simulink model "ddc_bpm_476_066"  (Simulink 7.8)
settings: Solver=ode45  StartTime=0.0  StopTime=2e-3  RelTol=1e-3
undefined symbols (not defined in the file): decim_factor_poly_35, dt_sim, frev_476, Fs_adc, n_ch, n_ovs, R_fofb, R_sec, R_sec_cfir, R_sec_pfir, xlipgetpartsetting
libraries: xbsIndex_r4 x1483, simulink x7
(part 11 of 12)

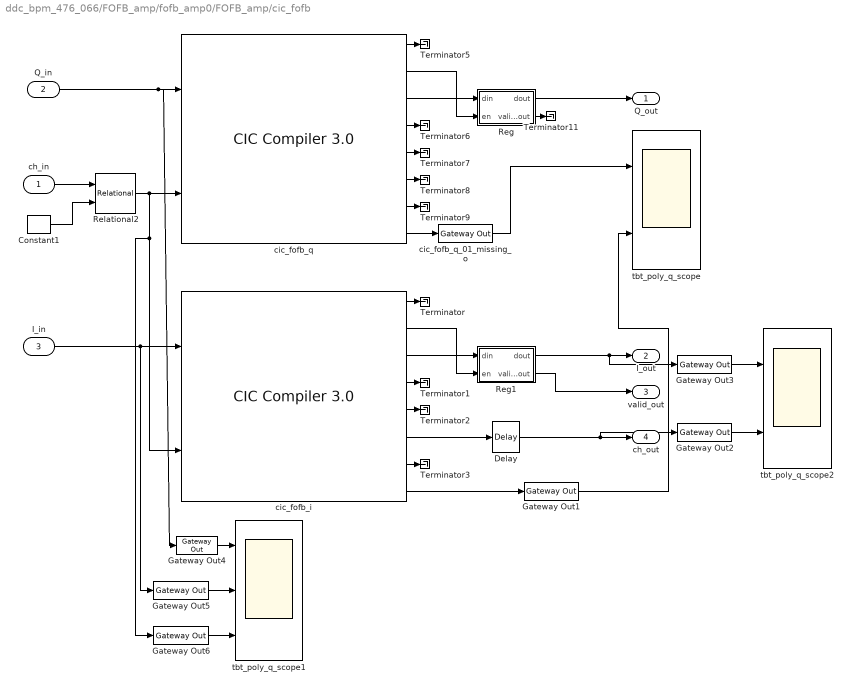
== system ddc_bpm_476_066/FOFB_amp/fofb_amp0/FOFB_amp/cic_fofb ==
  ch_in : Inport
  Q_in : Inport  Port=2
  I_in : Inport  Port=3
  Constant1 : xbsIndex_r4/Constant  const=0  gui_display_data_type=Fixed-point  arith_type=Unsigned  n_bits=2  bin_pt=0  preci_type=Single  exp_width=8  frac_width=24  explicit_period=off  period=1  equ=P=C  opselect=C  inp2=PCIN>>17  opr=+  inp1=P  carry=CIN  dbl_ovrd=off  block_type=constant
  Delay : xbsIndex_r4/Delay  rst=off  infoeditControl=Selection of Reset will increase slice count due to use of real FFs and instead of SRLs  en=off  latency=1  dbl_ovrd=off  reg_retiming=off  block_type=delay
  Gateway Out{1..6} (6 alike) : xbsIndex_r4/Gateway Out  inherit_from_input=on  hdl_port=off  timing_constraint=Data Rate  locs_specified=off  LOCs={}  UseAsDAC=off  DACChannel='1'  block_type=gatewayout
      settings: infoedit="Gateway out block.  Converts Xilinx fixed-point or floating-point type inputs into ouputs of type Simulink integer, single, double, or fixed point.<br><br>Hardware notes:  In hardware these blocks become top level output ports or are discarded, depending on how they are configured."
  Reg : Subsystem
  Reg1 : Subsystem
  Relational2 : xbsIndex_r4/Relational  mode=a=b  en=off  latency=1  dbl_ovrd=off  block_type=relational
  Terminator{,1..3,5..9,11} (10 alike) : Terminator
  cic_fofb_i : xbsIndex_r4/CIC Compiler 3.0   filter_type=Decimation  number_of_stages=5  differential_delay=2  number_of_channels=2  sample_rate_changes=Fixed  fixed_or_initial_rate=R_fofb  minimum_rate=1112  maximum_rate=1112  ratespecification=Maximum_Possible  sampleperiod=1  hardwareoversamplingrate=556  quantization=Full_Precision  output_data_width=74  use_xtreme_dsp_slice=on  use_streaming_interface=on  has_aclken=off  has_aresetn=off  has_dout_tready=off  trim_axipin_name=on  gui_behaviour=Sysgen_GUI  input_data_width=18  ip_name=CIC Compiler  ip_version=3.0  dsptool_ready=true  wrapper_available=true  port_translation_map={ 'aclken' => 'en', 'aresetn' => 'rst' }  ipcore_xco_need_fpga_part=true  ipcore_fpga_part=xlipgetpartsetting(gcb, {'virtex7', 'xc7v1500t', '-2', 'fhg1157'})  ipcore_verbose=false  block_type=cic_compiler_v3_0
  cic_fofb_q : xbsIndex_r4/CIC Compiler 3.0   filter_type=Decimation  number_of_stages=5  differential_delay=2  number_of_channels=2  sample_rate_changes=Fixed  fixed_or_initial_rate=R_fofb  minimum_rate=1112  maximum_rate=1112  ratespecification=Maximum_Possible  sampleperiod=1  hardwareoversamplingrate=556  quantization=Full_Precision  output_data_width=74  use_xtreme_dsp_slice=on  use_streaming_interface=on  has_aclken=off  has_aresetn=off  has_dout_tready=off  trim_axipin_name=on  gui_behaviour=Sysgen_GUI  input_data_width=18  ip_name=CIC Compiler  ip_version=3.0  dsptool_ready=true  wrapper_available=true  port_translation_map={ 'aclken' => 'en', 'aresetn' => 'rst' }  ipcore_xco_need_fpga_part=true  ipcore_fpga_part=xlipgetpartsetting(gcb, {'virtex7', 'xc7v1500t', '-2', 'fhg1157'})  ipcore_verbose=false  block_type=cic_compiler_v3_0
  cic_fofb_q_01_missing_o : xbsIndex_r4/Gateway Out  inherit_from_input=on  hdl_port=on  timing_constraint=Data Rate  locs_specified=off  LOCs={}  UseAsDAC=off  DACChannel='1'  block_type=gatewayout
      settings: infoedit="Gateway out block.  Converts Xilinx fixed-point or floating-point type inputs into ouputs of type Simulink integer, single, double, or fixed point.<br><br>Hardware notes:  In hardware these blocks become top level output ports or are discarded, depending on how they are configured."
  tbt_poly_q_scope : Scope  NumInputPorts=2
      settings: TimeRange=0.00011214  YMin=-0.1~-1.5  YMax=1~1.5  SaveName=ScopeData11  MaxDataPoints=1000000  SampleInput=on
  tbt_poly_q_scope1 : Scope  NumInputPorts=3
      settings: TimeRange=0.00011214  YMin=-0.1~-1.5~-5  YMax=1~1.5~5  SaveName=ScopeData12  MaxDataPoints=1000000  SampleInput=on
  tbt_poly_q_scope2 : Scope  NumInputPorts=2
      settings: TimeRange=0.00018  YMin=-5.05447e-005~0.9999999998750002  YMax=-5.05447e-005~1.000000000125  SaveName=ScopeData17  MaxDataPoints=1000000  SampleInput=on
  Q_out : Outport
  I_out : Outport  Port=2
  valid_out : Outport  Port=3
  ch_out : Outport  Port=4
  wires:
  I_in/1 -> cic_fofb_i/1, Gateway Out5/1
  Q_in/1 -> cic_fofb_q/1, Gateway Out4/1
  Relational2/1 -> cic_fofb_q/2, cic_fofb_i/2, Gateway Out6/1
  ch_in/1 -> Relational2/1
  cic_fofb_i/6 -> Delay/1
  cic_fofb_i/1 -> Terminator/1
  cic_fofb_i/4 -> Terminator1/1
  cic_fofb_i/5 -> Terminator2/1
  cic_fofb_i/7 -> Terminator3/1
  cic_fofb_q/1 -> Terminator5/1
  cic_fofb_q/4 -> Terminator6/1
  cic_fofb_q/5 -> Terminator7/1
  cic_fofb_q/6 -> Terminator8/1
  cic_fofb_q/7 -> Terminator9/1
  Constant1/1 -> Relational2/2
  Reg/1(dout) -> Q_out/1
  cic_fofb_q/3 -> Reg/1(din)
  cic_fofb_q/2 -> Reg/2(en)
  Reg1/1(dout) -> I_out/1, Gateway Out3/1
  cic_fofb_i/3 -> Reg1/1(din)
  cic_fofb_i/2 -> Reg1/2(en)
  Reg1/2(valid_out) -> valid_out/1
  Delay/1 -> ch_out/1, Gateway Out2/1
  Reg/2(valid_out) -> Terminator11/1
  cic_fofb_q/8 -> cic_fofb_q_01_missing_o/1
  cic_fofb_i/8 -> Gateway Out1/1
  cic_fofb_q_01_missing_o/1 -> tbt_poly_q_scope/1
  Gateway Out1/1 -> tbt_poly_q_scope/2
  Gateway Out2/1 -> tbt_poly_q_scope2/2
  Gateway Out3/1 -> tbt_poly_q_scope2/1
  Gateway Out4/1 -> tbt_poly_q_scope1/1
  Gateway Out5/1 -> tbt_poly_q_scope1/2
  Gateway Out6/1 -> tbt_poly_q_scope1/3

== system ddc_bpm_476_066/FOFB_amp/fofb_amp1/FOFB_CORDIC/TDDM_fofb_cordic1 ==
  fofb_cordic_din : Inport
  fofb_cordic_pin : Inport  Port=2
  fofb_cordic_ch_in : Inport  Port=3
  TDDM_fofb_cordic1_int : Subsystem
  TDDM_tbt_cordic1 : Subsystem
  Terminator : Terminator
  Terminator1 : Terminator
  fofb_cordic_data0_out : Outport
  fofb_cordic_data1_out : Outport  Port=2
  fofb_cordic_phase0_out : Outport  Port=3
  fofb_cordic_phase1_out : Outport  Port=4
  wires:
  TDDM_fofb_cordic1_int/2(dout_ch1) -> fofb_cordic_data1_out/1
  fofb_cordic_din/1 -> TDDM_fofb_cordic1_int/1(din)
  fofb_cordic_ch_in/1 -> TDDM_fofb_cordic1_int/2(ch_in), TDDM_tbt_cordic1/2(ch_in)
  TDDM_fofb_cordic1_int/1(dout_ch0) -> fofb_cordic_data0_out/1
  TDDM_fofb_cordic1_int/3(ch_out) -> Terminator/1
  TDDM_tbt_cordic1/2(dout_ch1) -> fofb_cordic_phase1_out/1
  fofb_cordic_pin/1 -> TDDM_tbt_cordic1/1(din)
  TDDM_tbt_cordic1/1(dout_ch0) -> fofb_cordic_phase0_out/1
  TDDM_tbt_cordic1/3(ch_out) -> Terminator1/1

== system ddc_bpm_476_066/FOFB_amp/fofb_amp1/FOFB_amp/Reg ==
  din : Inport
  Convert : xbsIndex_r4/Convert  gui_display_data_type=Fixed-point  arith_type="Signed  (2's comp)"  n_bits=24  bin_pt=22  float_type=Single  exp_bits=8  fraction_bits=24  quantization="Round  (unbiased: +/- Inf)"  overflow=Flag as error  en=off  latency=0  dbl_ovrd=off  pipeline=off  block_type=convert
  Register : xbsIndex_r4/Register  init=0  rst=off  en=off  dbl_ovrd=off  block_type=register
      settings: xl_area=[0, 0, 0, 0, 0, 0, 0]  block_version=VER_STRING_GOES_HERE
  Reinterpret2 : xbsIndex_r4/Reinterpret  force_arith_type=on  arith_type="Signed  (2's comp)"  force_bin_pt=on  bin_pt=23  block_type=cast
      settings: block_version=VER_STRING_GOES_HERE
  dout : Outport
  wires:
  Register/1 -> dout/1
  din/1 -> Reinterpret2/1
  Reinterpret2/1 -> Convert/1
  Convert/1 -> Register/1

== system ddc_bpm_476_066/FOFB_amp/fofb_amp1/FOFB_amp/Reg1 ==
  din : Inport
  Convert : xbsIndex_r4/Convert  gui_display_data_type=Fixed-point  arith_type="Signed  (2's comp)"  n_bits=24  bin_pt=22  float_type=Single  exp_bits=8  fraction_bits=24  quantization="Round  (unbiased: +/- Inf)"  overflow=Flag as error  en=off  latency=0  dbl_ovrd=off  pipeline=off  block_type=convert
  Register : xbsIndex_r4/Register  init=0  rst=off  en=off  dbl_ovrd=off  block_type=register
      settings: xl_area=[0, 0, 0, 0, 0, 0, 0]  block_version=VER_STRING_GOES_HERE
  Reinterpret2 : xbsIndex_r4/Reinterpret  force_arith_type=on  arith_type="Signed  (2's comp)"  force_bin_pt=on  bin_pt=23  block_type=cast
      settings: block_version=VER_STRING_GOES_HERE
  dout : Outport
  wires:
  Register/1 -> dout/1
  din/1 -> Reinterpret2/1
  Reinterpret2/1 -> Convert/1
  Convert/1 -> Register/1

== system ddc_bpm_476_066/FOFB_amp/fofb_amp1/FOFB_amp/TDDM_fofb_cic1 ==
  fofb_q_in : Inport
  fofb_i_in : Inport  Port=2
  fofb_ch_in : Inport  Port=3
  TDDM_fofb_cic1_i : Subsystem
  TDDM_fofb_cic1_q : Subsystem
  Terminator : Terminator
  Terminator1 : Terminator
  cic_fofb_ch0_q_out : Outport
  cic_fofb_ch1_q_out : Outport  Port=2
  cic_fofb_ch0_i_out : Outport  Port=3
  cic_fofb_ch1_i_out : Outport  Port=4
  wires:
  fofb_q_in/1 -> TDDM_fofb_cic1_q/1(din)
  fofb_ch_in/1 -> TDDM_fofb_cic1_q/2(ch_in), TDDM_fofb_cic1_i/2(ch_in)
  fofb_i_in/1 -> TDDM_fofb_cic1_i/1(din)
  TDDM_fofb_cic1_q/1(dout_ch0) -> cic_fofb_ch0_q_out/1
  TDDM_fofb_cic1_q/2(dout_ch1) -> cic_fofb_ch1_q_out/1
  TDDM_fofb_cic1_i/2(dout_ch1) -> cic_fofb_ch1_i_out/1
  TDDM_fofb_cic1_i/1(dout_ch0) -> cic_fofb_ch0_i_out/1
  TDDM_fofb_cic1_i/3(ch_out) -> Terminator/1
  TDDM_fofb_cic1_q/3(ch_out) -> Terminator1/1

== system ddc_bpm_476_066/FOFB_amp/fofb_amp1/FOFB_amp/cic_fofb ==
  ch_in : Inport
  Q_in : Inport  Port=2
  I_in : Inport  Port=3
  Constant1 : xbsIndex_r4/Constant  const=0  gui_display_data_type=Fixed-point  arith_type=Unsigned  n_bits=2  bin_pt=0  preci_type=Single  exp_width=8  frac_width=24  explicit_period=off  period=1  equ=P=C  opselect=C  inp2=PCIN>>17  opr=+  inp1=P  carry=CIN  dbl_ovrd=off  block_type=constant
  Delay : xbsIndex_r4/Delay  rst=off  infoeditControl=Selection of Reset will increase slice count due to use of real FFs and instead of SRLs  en=off  latency=1  dbl_ovrd=off  reg_retiming=off  block_type=delay
  Reg : Subsystem
  Reg1 : Subsystem
  Relational2 : xbsIndex_r4/Relational  mode=a=b  en=off  latency=1  dbl_ovrd=off  block_type=relational
  Terminator{,1..11} (12 alike) : Terminator
  cic_fofb_i : xbsIndex_r4/CIC Compiler 3.0   filter_type=Decimation  number_of_stages=5  differential_delay=2  number_of_channels=2  sample_rate_changes=Fixed  fixed_or_initial_rate=R_fofb  minimum_rate=1112  maximum_rate=1112  ratespecification=Maximum_Possible  sampleperiod=1  hardwareoversamplingrate=556  quantization=Full_Precision  output_data_width=74  use_xtreme_dsp_slice=on  use_streaming_interface=on  has_aclken=off  has_aresetn=off  has_dout_tready=off  trim_axipin_name=on  gui_behaviour=Sysgen_GUI  input_data_width=18  ip_name=CIC Compiler  ip_version=3.0  dsptool_ready=true  wrapper_available=true  port_translation_map={ 'aclken' => 'en', 'aresetn' => 'rst' }  ipcore_xco_need_fpga_part=true  ipcore_fpga_part=xlipgetpartsetting(gcb, {'virtex7', 'xc7v1500t', '-2', 'fhg1157'})  ipcore_verbose=false  block_type=cic_compiler_v3_0
  cic_fofb_q : xbsIndex_r4/CIC Compiler 3.0   filter_type=Decimation  number_of_stages=5  differential_delay=2  number_of_channels=2  sample_rate_changes=Fixed  fixed_or_initial_rate=R_fofb  minimum_rate=1112  maximum_rate=1112  ratespecification=Maximum_Possible  sampleperiod=1  hardwareoversamplingrate=556  quantization=Full_Precision  output_data_width=74  use_xtreme_dsp_slice=on  use_streaming_interface=on  has_aclken=off  has_aresetn=off  has_dout_tready=off  trim_axipin_name=on  gui_behaviour=Sysgen_GUI  input_data_width=18  ip_name=CIC Compiler  ip_version=3.0  dsptool_ready=true  wrapper_available=true  port_translation_map={ 'aclken' => 'en', 'aresetn' => 'rst' }  ipcore_xco_need_fpga_part=true  ipcore_fpga_part=xlipgetpartsetting(gcb, {'virtex7', 'xc7v1500t', '-2', 'fhg1157'})  ipcore_verbose=false  block_type=cic_compiler_v3_0
  cic_fofb_q_23_missing_o : xbsIndex_r4/Gateway Out  inherit_from_input=on  hdl_port=on  timing_constraint=Data Rate  locs_specified=off  LOCs={}  UseAsDAC=off  DACChannel='1'  block_type=gatewayout
      settings: infoedit="Gateway out block.  Converts Xilinx fixed-point or floating-point type inputs into ouputs of type Simulink integer, single, double, or fixed point.<br><br>Hardware notes:  In hardware these blocks become top level output ports or are discarded, depending on how they are configured."
  Q_out : Outport
  I_out : Outport  Port=2
  valid_out : Outport  Port=3
  ch_out : Outport  Port=4
  wires:
  I_in/1 -> cic_fofb_i/1
  Q_in/1 -> cic_fofb_q/1
  Relational2/1 -> cic_fofb_q/2, cic_fofb_i/2
  ch_in/1 -> Relational2/1
  cic_fofb_i/1 -> Terminator/1
  cic_fofb_i/4 -> Terminator1/1
  cic_fofb_i/5 -> Terminator2/1
  cic_fofb_i/7 -> Terminator3/1
  cic_fofb_i/8 -> Terminator4/1
  cic_fofb_q/1 -> Terminator5/1
  cic_fofb_q/4 -> Terminator6/1
  cic_fofb_q/5 -> Terminator7/1
  cic_fofb_q/6 -> Terminator8/1
  cic_fofb_q/7 -> Terminator9/1
  cic_fofb_q/8 -> cic_fofb_q_23_missing_o/1
  Constant1/1 -> Relational2/2
  Reg/1(dout) -> Q_out/1
  cic_fofb_q/3 -> Reg/1(din)
  cic_fofb_q/2 -> Reg/2(en)
  Reg1/1(dout) -> I_out/1
  cic_fofb_i/3 -> Reg1/1(din)
  cic_fofb_i/2 -> Reg1/2(en)
  Delay/1 -> ch_out/1
  cic_fofb_i/6 -> Delay/1
  Reg1/2(valid_out) -> valid_out/1
  Reg/2(valid_out) -> Terminator11/1
  cic_fofb_q_23_missing_o/1 -> Terminator10/1

== system ddc_bpm_476_066/Monit_amp/Monit_amp_c/Cast2/format1 ==
  din : Inport
  Convert : xbsIndex_r4/Convert  gui_display_data_type=Fixed-point  arith_type="Signed  (2's comp)"  n_bits=24  bin_pt=22  float_type=Single  exp_bits=8  fraction_bits=24  quantization="Round  (unbiased: +/- Inf)"  overflow=Flag as error  en=off  latency=0  dbl_ovrd=off  pipeline=off  block_type=convert
  Reinterpret : xbsIndex_r4/Reinterpret  force_arith_type=on  arith_type="Signed  (2's comp)"  force_bin_pt=off  bin_pt=22  block_type=reinterpret
      settings: block_version=10.1
  dout : Outport
  wires:
  din/1 -> Reinterpret/1
  Convert/1 -> dout/1
  Reinterpret/1 -> Convert/1

== system ddc_bpm_476_066/Monit_amp/Monit_amp_c/Cast4/format1 ==
  din : Inport
  Convert : xbsIndex_r4/Convert  gui_display_data_type=Fixed-point  arith_type="Signed  (2's comp)"  n_bits=24  bin_pt=22  float_type=Single  exp_bits=8  fraction_bits=24  quantization="Round  (unbiased: +/- Inf)"  overflow=Flag as error  en=off  latency=0  dbl_ovrd=off  pipeline=off  block_type=convert
  Reinterpret : xbsIndex_r4/Reinterpret  force_arith_type=on  arith_type="Signed  (2's comp)"  force_bin_pt=off  bin_pt=22  block_type=reinterpret
      settings: block_version=10.1
  dout : Outport
  wires:
  din/1 -> Reinterpret/1
  Reinterpret/1 -> Convert/1
  Convert/1 -> dout/1

== system ddc_bpm_476_066/Monit_amp/Monit_amp_c/TDDM_monit_amp_c/TDDM_monit_amp_c_int ==
  din : Inport
  ch_in : Inport  Port=2
  Constant : xbsIndex_r4/Constant  const=3  gui_display_data_type=Fixed-point  arith_type=Unsigned  n_bits=2  bin_pt=0  preci_type=Single  exp_width=8  frac_width=24  explicit_period=off  period=1  equ=P=C  opselect=C  inp2=PCIN>>17  opr=+  inp1=P  carry=CIN  dbl_ovrd=off  block_type=constant
  Constant1 : xbsIndex_r4/Constant  const=0  gui_display_data_type=Fixed-point  arith_type=Unsigned  n_bits=2  bin_pt=0  preci_type=Single  exp_width=8  frac_width=24  explicit_period=off  period=1  equ=P=C  opselect=C  inp2=PCIN>>17  opr=+  inp1=P  carry=CIN  dbl_ovrd=off  block_type=constant
  Constant3 : xbsIndex_r4/Constant  const=1  gui_display_data_type=Fixed-point  arith_type=Unsigned  n_bits=2  bin_pt=0  preci_type=Single  exp_width=8  frac_width=24  explicit_period=off  period=1  equ=P=C  opselect=C  inp2=PCIN>>17  opr=+  inp1=P  carry=CIN  dbl_ovrd=off  block_type=constant
  Constant4 : xbsIndex_r4/Constant  const=2  gui_display_data_type=Fixed-point  arith_type=Unsigned  n_bits=2  bin_pt=0  preci_type=Single  exp_width=8  frac_width=24  explicit_period=off  period=1  equ=P=C  opselect=C  inp2=PCIN>>17  opr=+  inp1=P  carry=CIN  dbl_ovrd=off  block_type=constant
  Delay : xbsIndex_r4/Delay  rst=off  infoeditControl=Selection of Reset will increase slice count due to use of real FFs and instead of SRLs  en=off  latency=3  dbl_ovrd=off  reg_retiming=off  block_type=delay
  Down Sample{1..4} (4 alike) : xbsIndex_r4/Down Sample  sample_ratio=n_ch  sample_phase="Last Value of Frame  (most efficient)"  en=off  latency=1  dbl_ovrd=off  block_type=dsamp
  Register{,1..3} (4 alike) : xbsIndex_r4/Register  init=0  rst=off  en=on  dbl_ovrd=off  block_type=register
  Relational{,1..3} (4 alike) : xbsIndex_r4/Relational  mode=a=b  en=off  latency=1  dbl_ovrd=off  block_type=relational
  dout_ch0 : Outport
  dout_ch1 : Outport  Port=2
  dout_ch2 : Outport  Port=3
  dout_ch3 : Outport  Port=4
  ch_out : Outport  Port=5
  wires:
  Constant/1 -> Relational/2
  Constant1/1 -> Relational1/2
  Constant3/1 -> Relational2/2
  Constant4/1 -> Relational3/2
  Relational/1 -> Register/2
  Relational1/1 -> Register1/2
  Relational2/1 -> Register2/2
  Relational3/1 -> Register3/2
  din/1 -> Register1/1, Register2/1, Register3/1, Register/1
  Register/1 -> Down Sample2/1
  ch_in/1 -> Relational/1, Relational1/1, Relational2/1, Relational3/1, Delay/1
  Register1/1 -> Down Sample1/1
  Register2/1 -> Down Sample3/1
  Register3/1 -> Down Sample4/1
  Down Sample2/1 -> dout_ch0/1
  Delay/1 -> ch_out/1
  Down Sample3/1 -> dout_ch2/1
  Down Sample1/1 -> dout_ch1/1
  Down Sample4/1 -> dout_ch3/1

== system ddc_bpm_476_066/TBT_amp/TBT_amp0/TBT_CORDIC/TDDM_tbt_cordic ==
  tbt_cordic_din : Inport
  tbt_cordic_pin : Inport  Port=2
  tbt_cordic_ch_in : Inport  Port=3
  TDDM_tbt_cordic : Subsystem
  TDDM_tbt_cordic1 : Subsystem
  Terminator : Terminator
  Terminator1 : Terminator
  tbt_cordic_data0_out : Outport
  tbt_cordic_data1_out : Outport  Port=2
  tbt_cordic_phase0_out : Outport  Port=3
  tbt_cordic_phase1_out : Outport  Port=4
  wires:
  TDDM_tbt_cordic/2(dout_ch1) -> tbt_cordic_data1_out/1
  tbt_cordic_din/1 -> TDDM_tbt_cordic/1(din)
  tbt_cordic_ch_in/1 -> TDDM_tbt_cordic/2(ch_in), TDDM_tbt_cordic1/2(ch_in)
  TDDM_tbt_cordic/1(dout_ch0) -> tbt_cordic_data0_out/1
  TDDM_tbt_cordic/3(ch_out) -> Terminator/1
  TDDM_tbt_cordic1/2(dout_ch1) -> tbt_cordic_phase1_out/1
  tbt_cordic_pin/1 -> TDDM_tbt_cordic1/1(din)
  TDDM_tbt_cordic1/1(dout_ch0) -> tbt_cordic_phase0_out/1
  TDDM_tbt_cordic1/3(ch_out) -> Terminator1/1

== system ddc_bpm_476_066/TBT_amp/TBT_amp0/TBT_poly_decim/ST3 ==
  In : Inport
  Display : Display
  Sample Time : xbsIndex_r4/Sample Time  block_type=sampletime
      settings: infoedit="The Sample Time block reports the normalized sample period of its input.  A signal's normalized sample period is not equivalent to its Simulink absolute sample period.<br><br>Hardware notes: This block is implemented as a constant in hardware."
  out : xbsIndex_r4/Gateway Out  inherit_from_input=on  hdl_port=off  timing_constraint=Data Rate  locs_specified=off  LOCs={}  UseAsDAC=off  DACChannel='1'  block_type=gatewayout
      settings: infoedit="Gateway out block.  Converts Xilinx fixed-point or floating-point type inputs into ouputs of type Simulink integer, single, double, or fixed point.<br><br>Hardware notes:  In hardware these blocks become top level output ports or are discarded, depending on how they are configured."
  wires:
  out/1 -> Display/1
  Sample Time/1 -> out/1
  In/1 -> Sample Time/1

== system ddc_bpm_476_066/TBT_amp/TBT_amp0/TBT_poly_decim/TDDM_TBT ==
  tbt_q_in : Inport
  tbt_i_in : Inport  Port=2
  tbt_ch_in : Inport  Port=3
  TDDM_tbt_poly_i : Subsystem
  TDDM_tbt_poly_q : Subsystem
  Terminator : Terminator
  Terminator1 : Terminator
  poly35_ch0_q_out : Outport
  poly35_ch1_q_out : Outport  Port=2
  poly35_ch0_i_out : Outport  Port=3
  poly35_ch1_i_out : Outport  Port=4
  wires:
  tbt_q_in/1 -> TDDM_tbt_poly_q/1(din)
  tbt_ch_in/1 -> TDDM_tbt_poly_q/2(ch_in), TDDM_tbt_poly_i/2(ch_in)
  tbt_i_in/1 -> TDDM_tbt_poly_i/1(din)
  TDDM_tbt_poly_q/1(dout_ch0) -> poly35_ch0_q_out/1
  TDDM_tbt_poly_q/2(dout_ch1) -> poly35_ch1_q_out/1
  TDDM_tbt_poly_i/2(dout_ch1) -> poly35_ch1_i_out/1
  TDDM_tbt_poly_i/1(dout_ch0) -> poly35_ch0_i_out/1
  TDDM_tbt_poly_i/3(ch_out) -> Terminator/1
  TDDM_tbt_poly_q/3(ch_out) -> Terminator1/1

== system ddc_bpm_476_066/TBT_amp/TBT_amp0/TBT_poly_decim/Trunc ==
  din : Inport
  Reinterpret : xbsIndex_r4/Reinterpret  force_arith_type=on  arith_type="Signed  (2's comp)"  force_bin_pt=on  bin_pt=22  block_type=reinterpret
  Slice : xbsIndex_r4/Slice  nbits=24  boolean_output=off  mode=Upper Bit Location + Width  bit1=0  base1=MSB of Input  bit0=0  base0=LSB of Input  dbl_ovrd=off  block_type=slice
  dout : Outport
  wires:
  Slice/1 -> Reinterpret/1
  Reinterpret/1 -> dout/1
  din/1 -> Slice/1

== system ddc_bpm_476_066/TBT_amp/TBT_amp0/TBT_poly_decim/Trunc1 ==
  din : Inport
  Reinterpret : xbsIndex_r4/Reinterpret  force_arith_type=on  arith_type="Signed  (2's comp)"  force_bin_pt=on  bin_pt=22  block_type=reinterpret
  Slice : xbsIndex_r4/Slice  nbits=24  boolean_output=off  mode=Upper Bit Location + Width  bit1=0  base1=MSB of Input  bit0=0  base0=LSB of Input  dbl_ovrd=off  block_type=slice
  dout : Outport
  wires:
  Slice/1 -> Reinterpret/1
  Reinterpret/1 -> dout/1
  din/1 -> Slice/1

== system ddc_bpm_476_066/TBT_amp/TBT_amp1/TBT_CORDIC/TDDM_tbt_cordic ==
  tbt_cordic_din : Inport
  tbt_cordic_pin : Inport  Port=2
  tbt_cordic_ch_in : Inport  Port=3
  TDDM_tbt_cordic : Subsystem
  TDDM_tbt_cordic1 : Subsystem
  Terminator : Terminator
  Terminator1 : Terminator
  tbt_cordic_ch2_out : Outport
  tbt_cordic_ch3_out : Outport  Port=2
  tbt_cordic_phase0_out : Outport  Port=3
  tbt_cordic_phase1_out : Outport  Port=4
  wires:
  TDDM_tbt_cordic/2(dout_ch1) -> tbt_cordic_ch3_out/1
  tbt_cordic_din/1 -> TDDM_tbt_cordic/1(din)
  tbt_cordic_ch_in/1 -> TDDM_tbt_cordic/2(ch_in), TDDM_tbt_cordic1/2(ch_in)
  TDDM_tbt_cordic/1(dout_ch0) -> tbt_cordic_ch2_out/1
  TDDM_tbt_cordic/3(ch_out) -> Terminator/1
  TDDM_tbt_cordic1/2(dout_ch1) -> tbt_cordic_phase1_out/1
  tbt_cordic_pin/1 -> TDDM_tbt_cordic1/1(din)
  TDDM_tbt_cordic1/1(dout_ch0) -> tbt_cordic_phase0_out/1
  TDDM_tbt_cordic1/3(ch_out) -> Terminator1/1

== system ddc_bpm_476_066/TBT_amp/TBT_amp1/TBT_poly_decim/TDDM_TBT ==
  tbt_q_in : Inport
  tbt_i_in : Inport  Port=2
  tbt_ch_in : Inport  Port=3
  TDDM_tbt_poly_i : Subsystem
  TDDM_tbt_poly_q : Subsystem
  Terminator : Terminator
  Terminator1 : Terminator
  poly35_ch2_q_out : Outport
  poly35_ch3_q_out : Outport  Port=2
  poly35_ch2_i_out : Outport  Port=3
  poly35_ch3_i_out : Outport  Port=4
  wires:
  tbt_q_in/1 -> TDDM_tbt_poly_q/1(din)
  tbt_ch_in/1 -> TDDM_tbt_poly_q/2(ch_in), TDDM_tbt_poly_i/2(ch_in)
  tbt_i_in/1 -> TDDM_tbt_poly_i/1(din)
  TDDM_tbt_poly_q/1(dout_ch0) -> poly35_ch2_q_out/1
  TDDM_tbt_poly_q/2(dout_ch1) -> poly35_ch3_q_out/1
  TDDM_tbt_poly_i/2(dout_ch1) -> poly35_ch3_i_out/1
  TDDM_tbt_poly_i/1(dout_ch0) -> poly35_ch2_i_out/1
  TDDM_tbt_poly_i/3(ch_out) -> Terminator/1
  TDDM_tbt_poly_q/3(ch_out) -> Terminator1/1

== system ddc_bpm_476_066/TBT_amp/TBT_amp1/TBT_poly_decim/Trunc ==
  din : Inport
  Reinterpret : xbsIndex_r4/Reinterpret  force_arith_type=on  arith_type="Signed  (2's comp)"  force_bin_pt=on  bin_pt=22  block_type=reinterpret
  Slice : xbsIndex_r4/Slice  nbits=24  boolean_output=off  mode=Upper Bit Location + Width  bit1=0  base1=MSB of Input  bit0=0  base0=LSB of Input  dbl_ovrd=off  block_type=slice
  dout : Outport
  wires:
  Slice/1 -> Reinterpret/1
  Reinterpret/1 -> dout/1
  din/1 -> Slice/1

== system ddc_bpm_476_066/TBT_amp/TBT_amp1/TBT_poly_decim/Trunc1 ==
  din : Inport
  Reinterpret : xbsIndex_r4/Reinterpret  force_arith_type=on  arith_type="Signed  (2's comp)"  force_bin_pt=on  bin_pt=22  block_type=reinterpret
  Slice : xbsIndex_r4/Slice  nbits=24  boolean_output=off  mode=Upper Bit Location + Width  bit1=0  base1=MSB of Input  bit0=0  base0=LSB of Input  dbl_ovrd=off  block_type=slice
  dout : Outport
  wires:
  Slice/1 -> Reinterpret/1
  Reinterpret/1 -> dout/1
  din/1 -> Slice/1

== system ddc_bpm_476_066/FOFB_amp/fofb_amp0/FOFB_CORDIC/TDDM_tbt_cordic0/TDDM_fofb_cordic0_int ==
  din : Inport
  ch_in : Inport  Port=2
  Constant : xbsIndex_r4/Constant  const=1  gui_display_data_type=Fixed-point  arith_type=Unsigned  n_bits=1  bin_pt=0  preci_type=Single  exp_width=8  frac_width=24  explicit_period=off  period=1  equ=P=C  opselect=C  inp2=PCIN>>17  opr=+  inp1=P  carry=CIN  dbl_ovrd=off  block_type=constant
  Constant1 : xbsIndex_r4/Constant  const=0  gui_display_data_type=Fixed-point  arith_type=Unsigned  n_bits=1  bin_pt=0  preci_type=Single  exp_width=8  frac_width=24  explicit_period=off  period=1  equ=P=C  opselect=C  inp2=PCIN>>17  opr=+  inp1=P  carry=CIN  dbl_ovrd=off  block_type=constant
  Delay : xbsIndex_r4/Delay  rst=off  infoeditControl=Selection of Reset will increase slice count due to use of real FFs and instead of SRLs  en=off  latency=3  dbl_ovrd=off  reg_retiming=off  block_type=delay
  Down Sample1 : xbsIndex_r4/Down Sample  sample_ratio=n_ch/n_ovs  sample_phase="Last Value of Frame  (most efficient)"  en=off  latency=1  dbl_ovrd=off  block_type=dsamp
  Down Sample2 : xbsIndex_r4/Down Sample  sample_ratio=n_ch/n_ovs  sample_phase="Last Value of Frame  (most efficient)"  en=off  latency=1  dbl_ovrd=off  block_type=dsamp
  Register : xbsIndex_r4/Register  init=0  rst=off  en=on  dbl_ovrd=off  block_type=register
  Register1 : xbsIndex_r4/Register  init=0  rst=off  en=on  dbl_ovrd=off  block_type=register
  Relational : xbsIndex_r4/Relational  mode=a=b  en=off  latency=1  dbl_ovrd=off  block_type=relational
  Relational1 : xbsIndex_r4/Relational  mode=a=b  en=off  latency=1  dbl_ovrd=off  block_type=relational
  dout_ch0 : Outport
  dout_ch1 : Outport  Port=2
  ch_out : Outport  Port=3
  wires:
  Constant/1 -> Relational/2
  Constant1/1 -> Relational1/2
  Relational/1 -> Register/2
  Relational1/1 -> Register1/2
  din/1 -> Register/1, Register1/1
  Register/1 -> Down Sample2/1
  ch_in/1 -> Relational/1, Relational1/1, Delay/1
  Register1/1 -> Down Sample1/1
  Down Sample2/1 -> dout_ch0/1
  Delay/1 -> ch_out/1
  Down Sample1/1 -> dout_ch1/1

== system ddc_bpm_476_066/FOFB_amp/fofb_amp0/FOFB_CORDIC/TDDM_tbt_cordic0/TDDM_tbt_cordic1 ==
  din : Inport
  ch_in : Inport  Port=2
  Constant : xbsIndex_r4/Constant  const=1  gui_display_data_type=Fixed-point  arith_type=Unsigned  n_bits=1  bin_pt=0  preci_type=Single  exp_width=8  frac_width=24  explicit_period=off  period=1  equ=P=C  opselect=C  inp2=PCIN>>17  opr=+  inp1=P  carry=CIN  dbl_ovrd=off  block_type=constant
  Constant1 : xbsIndex_r4/Constant  const=0  gui_display_data_type=Fixed-point  arith_type=Unsigned  n_bits=1  bin_pt=0  preci_type=Single  exp_width=8  frac_width=24  explicit_period=off  period=1  equ=P=C  opselect=C  inp2=PCIN>>17  opr=+  inp1=P  carry=CIN  dbl_ovrd=off  block_type=constant
  Delay : xbsIndex_r4/Delay  rst=off  infoeditControl=Selection of Reset will increase slice count due to use of real FFs and instead of SRLs  en=off  latency=3  dbl_ovrd=off  reg_retiming=off  block_type=delay
  Down Sample1 : xbsIndex_r4/Down Sample  sample_ratio=n_ch/n_ovs  sample_phase="Last Value of Frame  (most efficient)"  en=off  latency=1  dbl_ovrd=off  block_type=dsamp
  Down Sample2 : xbsIndex_r4/Down Sample  sample_ratio=n_ch/n_ovs  sample_phase="Last Value of Frame  (most efficient)"  en=off  latency=1  dbl_ovrd=off  block_type=dsamp
  Register : xbsIndex_r4/Register  init=0  rst=off  en=on  dbl_ovrd=off  block_type=register
  Register1 : xbsIndex_r4/Register  init=0  rst=off  en=on  dbl_ovrd=off  block_type=register
  Relational : xbsIndex_r4/Relational  mode=a=b  en=off  latency=1  dbl_ovrd=off  block_type=relational
  Relational1 : xbsIndex_r4/Relational  mode=a=b  en=off  latency=1  dbl_ovrd=off  block_type=relational
  dout_ch0 : Outport
  dout_ch1 : Outport  Port=2
  ch_out : Outport  Port=3
  wires:
  Constant/1 -> Relational/2
  Constant1/1 -> Relational1/2
  Relational/1 -> Register/2
  Relational1/1 -> Register1/2
  din/1 -> Register/1, Register1/1
  Register/1 -> Down Sample2/1
  ch_in/1 -> Relational/1, Relational1/1, Delay/1
  Register1/1 -> Down Sample1/1
  Down Sample2/1 -> dout_ch0/1
  Delay/1 -> ch_out/1
  Down Sample1/1 -> dout_ch1/1

== system ddc_bpm_476_066/FOFB_amp/fofb_amp0/FOFB_amp/TDDM_fofb_cic0/TDDM_fofb_cic0_i ==
  din : Inport
  ch_in : Inport  Port=2
  Constant : xbsIndex_r4/Constant  const=1  gui_display_data_type=Fixed-point  arith_type=Unsigned  n_bits=1  bin_pt=0  preci_type=Single  exp_width=8  frac_width=24  explicit_period=off  period=1  equ=P=C  opselect=C  inp2=PCIN>>17  opr=+  inp1=P  carry=CIN  dbl_ovrd=off  block_type=constant
  Constant1 : xbsIndex_r4/Constant  const=0  gui_display_data_type=Fixed-point  arith_type=Unsigned  n_bits=1  bin_pt=0  preci_type=Single  exp_width=8  frac_width=24  explicit_period=off  period=1  equ=P=C  opselect=C  inp2=PCIN>>17  opr=+  inp1=P  carry=CIN  dbl_ovrd=off  block_type=constant
  Delay : xbsIndex_r4/Delay  rst=off  infoeditControl=Selection of Reset will increase slice count due to use of real FFs and instead of SRLs  en=off  latency=3  dbl_ovrd=off  reg_retiming=off  block_type=delay
  Down Sample1 : xbsIndex_r4/Down Sample  sample_ratio=n_ch/n_ovs  sample_phase="Last Value of Frame  (most efficient)"  en=off  latency=1  dbl_ovrd=off  block_type=dsamp
  Down Sample2 : xbsIndex_r4/Down Sample  sample_ratio=n_ch/n_ovs  sample_phase="Last Value of Frame  (most efficient)"  en=off  latency=1  dbl_ovrd=off  block_type=dsamp
  Register : xbsIndex_r4/Register  init=0  rst=off  en=on  dbl_ovrd=off  block_type=register
  Register1 : xbsIndex_r4/Register  init=0  rst=off  en=on  dbl_ovrd=off  block_type=register
  Relational : xbsIndex_r4/Relational  mode=a=b  en=off  latency=1  dbl_ovrd=off  block_type=relational
  Relational1 : xbsIndex_r4/Relational  mode=a=b  en=off  latency=1  dbl_ovrd=off  block_type=relational
  dout_ch0 : Outport
  dout_ch1 : Outport  Port=2
  ch_out : Outport  Port=3
  wires:
  Constant/1 -> Relational/2
  Constant1/1 -> Relational1/2
  Relational/1 -> Register/2
  Relational1/1 -> Register1/2
  din/1 -> Register/1, Register1/1
  Register/1 -> Down Sample2/1
  ch_in/1 -> Relational/1, Relational1/1, Delay/1
  Register1/1 -> Down Sample1/1
  Down Sample2/1 -> dout_ch0/1
  Delay/1 -> ch_out/1
  Down Sample1/1 -> dout_ch1/1

== system ddc_bpm_476_066/FOFB_amp/fofb_amp0/FOFB_amp/TDDM_fofb_cic0/TDDM_fofb_cic0_q ==
  din : Inport
  ch_in : Inport  Port=2
  Constant : xbsIndex_r4/Constant  const=1  gui_display_data_type=Fixed-point  arith_type=Unsigned  n_bits=1  bin_pt=0  preci_type=Single  exp_width=8  frac_width=24  explicit_period=off  period=1  equ=P=C  opselect=C  inp2=PCIN>>17  opr=+  inp1=P  carry=CIN  dbl_ovrd=off  block_type=constant
  Constant1 : xbsIndex_r4/Constant  const=0  gui_display_data_type=Fixed-point  arith_type=Unsigned  n_bits=1  bin_pt=0  preci_type=Single  exp_width=8  frac_width=24  explicit_period=off  period=1  equ=P=C  opselect=C  inp2=PCIN>>17  opr=+  inp1=P  carry=CIN  dbl_ovrd=off  block_type=constant
  Delay : xbsIndex_r4/Delay  rst=off  infoeditControl=Selection of Reset will increase slice count due to use of real FFs and instead of SRLs  en=off  latency=3  dbl_ovrd=off  reg_retiming=off  block_type=delay
  Down Sample1 : xbsIndex_r4/Down Sample  sample_ratio=n_ch/n_ovs  sample_phase="Last Value of Frame  (most efficient)"  en=off  latency=1  dbl_ovrd=off  block_type=dsamp
  Down Sample2 : xbsIndex_r4/Down Sample  sample_ratio=n_ch/n_ovs  sample_phase="Last Value of Frame  (most efficient)"  en=off  latency=1  dbl_ovrd=off  block_type=dsamp
  Register : xbsIndex_r4/Register  init=0  rst=off  en=on  dbl_ovrd=off  block_type=register
  Register1 : xbsIndex_r4/Register  init=0  rst=off  en=on  dbl_ovrd=off  block_type=register
  Relational : xbsIndex_r4/Relational  mode=a=b  en=off  latency=1  dbl_ovrd=off  block_type=relational
  Relational1 : xbsIndex_r4/Relational  mode=a=b  en=off  latency=1  dbl_ovrd=off  block_type=relational
  dout_ch0 : Outport
  dout_ch1 : Outport  Port=2
  ch_out : Outport  Port=3
  wires:
  Constant/1 -> Relational/2
  Constant1/1 -> Relational1/2
  Relational/1 -> Register/2
  Relational1/1 -> Register1/2
  din/1 -> Register/1, Register1/1
  Register/1 -> Down Sample2/1
  ch_in/1 -> Relational/1, Relational1/1, Delay/1
  Register1/1 -> Down Sample1/1
  Down Sample2/1 -> dout_ch0/1
  Delay/1 -> ch_out/1
  Down Sample1/1 -> dout_ch1/1

== system ddc_bpm_476_066/FOFB_amp/fofb_amp0/FOFB_amp/cic_fofb/Reg ==
  din : Inport
  en : Inport  Port=2
  Convert : xbsIndex_r4/Convert  gui_display_data_type=Fixed-point  arith_type="Signed  (2's comp)"  n_bits=25  bin_pt=23  float_type=Single  exp_bits=8  fraction_bits=24  quantization="Round  (unbiased: +/- Inf)"  overflow=Flag as error  en=off  latency=0  dbl_ovrd=off  pipeline=off  block_type=convert
  Register : xbsIndex_r4/Register  init=0  rst=off  en=on  dbl_ovrd=off  block_type=register
      settings: xl_area=[0, 0, 0, 0, 0, 0, 0]  block_version=VER_STRING_GOES_HERE
  Register1 : xbsIndex_r4/Register  init=0  rst=off  en=off  dbl_ovrd=off  block_type=register
      settings: xl_area=[0, 0, 0, 0, 0, 0, 0]  block_version=VER_STRING_GOES_HERE
  Reinterpret2 : xbsIndex_r4/Reinterpret  force_arith_type=on  arith_type="Signed  (2's comp)"  force_bin_pt=on  bin_pt=77  block_type=cast
      settings: block_version=VER_STRING_GOES_HERE
  dout : Outport
  valid_out : Outport  Port=2
  wires:
  Register/1 -> dout/1
  en/1 -> Register/2, Register1/1
  din/1 -> Reinterpret2/1
  Reinterpret2/1 -> Convert/1
  Register1/1 -> valid_out/1
  Convert/1 -> Register/1

== system ddc_bpm_476_066/FOFB_amp/fofb_amp0/FOFB_amp/cic_fofb/Reg1 ==
  din : Inport
  en : Inport  Port=2
  Convert : xbsIndex_r4/Convert  gui_display_data_type=Fixed-point  arith_type="Signed  (2's comp)"  n_bits=25  bin_pt=23  float_type=Single  exp_bits=8  fraction_bits=24  quantization="Round  (unbiased: +/- Inf)"  overflow=Flag as error  en=off  latency=0  dbl_ovrd=off  pipeline=off  block_type=convert
  Register : xbsIndex_r4/Register  init=0  rst=off  en=on  dbl_ovrd=off  block_type=register
      settings: xl_area=[0, 0, 0, 0, 0, 0, 0]  block_version=VER_STRING_GOES_HERE
  Register1 : xbsIndex_r4/Register  init=0  rst=off  en=off  dbl_ovrd=off  block_type=register
      settings: xl_area=[0, 0, 0, 0, 0, 0, 0]  block_version=VER_STRING_GOES_HERE
  Reinterpret2 : xbsIndex_r4/Reinterpret  force_arith_type=on  arith_type="Signed  (2's comp)"  force_bin_pt=on  bin_pt=77  block_type=cast
      settings: block_version=VER_STRING_GOES_HERE
  dout : Outport
  valid_out : Outport  Port=2
  wires:
  Register/1 -> dout/1
  en/1 -> Register/2, Register1/1
  din/1 -> Reinterpret2/1
  Reinterpret2/1 -> Convert/1
  Register1/1 -> valid_out/1
  Convert/1 -> Register/1

== system ddc_bpm_476_066/FOFB_amp/fofb_amp1/FOFB_CORDIC/TDDM_fofb_cordic1/TDDM_fofb_cordic1_int ==
  din : Inport
  ch_in : Inport  Port=2
  Constant : xbsIndex_r4/Constant  const=1  gui_display_data_type=Fixed-point  arith_type=Unsigned  n_bits=1  bin_pt=0  preci_type=Single  exp_width=8  frac_width=24  explicit_period=off  period=1  equ=P=C  opselect=C  inp2=PCIN>>17  opr=+  inp1=P  carry=CIN  dbl_ovrd=off  block_type=constant
  Constant1 : xbsIndex_r4/Constant  const=0  gui_display_data_type=Fixed-point  arith_type=Unsigned  n_bits=1  bin_pt=0  preci_type=Single  exp_width=8  frac_width=24  explicit_period=off  period=1  equ=P=C  opselect=C  inp2=PCIN>>17  opr=+  inp1=P  carry=CIN  dbl_ovrd=off  block_type=constant
  Delay : xbsIndex_r4/Delay  rst=off  infoeditControl=Selection of Reset will increase slice count due to use of real FFs and instead of SRLs  en=off  latency=3  dbl_ovrd=off  reg_retiming=off  block_type=delay
  Down Sample1 : xbsIndex_r4/Down Sample  sample_ratio=n_ch/n_ovs  sample_phase="Last Value of Frame  (most efficient)"  en=off  latency=1  dbl_ovrd=off  block_type=dsamp
  Down Sample2 : xbsIndex_r4/Down Sample  sample_ratio=n_ch/n_ovs  sample_phase="Last Value of Frame  (most efficient)"  en=off  latency=1  dbl_ovrd=off  block_type=dsamp
  Register : xbsIndex_r4/Register  init=0  rst=off  en=on  dbl_ovrd=off  block_type=register
  Register1 : xbsIndex_r4/Register  init=0  rst=off  en=on  dbl_ovrd=off  block_type=register
  Relational : xbsIndex_r4/Relational  mode=a=b  en=off  latency=1  dbl_ovrd=off  block_type=relational
  Relational1 : xbsIndex_r4/Relational  mode=a=b  en=off  latency=1  dbl_ovrd=off  block_type=relational
  dout_ch0 : Outport
  dout_ch1 : Outport  Port=2
  ch_out : Outport  Port=3
  wires:
  Constant/1 -> Relational/2
  Constant1/1 -> Relational1/2
  Relational/1 -> Register/2
  Relational1/1 -> Register1/2
  din/1 -> Register/1, Register1/1
  Register/1 -> Down Sample2/1
  ch_in/1 -> Relational/1, Relational1/1, Delay/1
  Register1/1 -> Down Sample1/1
  Down Sample2/1 -> dout_ch0/1
  Delay/1 -> ch_out/1
  Down Sample1/1 -> dout_ch1/1

== system ddc_bpm_476_066/FOFB_amp/fofb_amp1/FOFB_CORDIC/TDDM_fofb_cordic1/TDDM_tbt_cordic1 ==
  din : Inport
  ch_in : Inport  Port=2
  Constant : xbsIndex_r4/Constant  const=1  gui_display_data_type=Fixed-point  arith_type=Unsigned  n_bits=1  bin_pt=0  preci_type=Single  exp_width=8  frac_width=24  explicit_period=off  period=1  equ=P=C  opselect=C  inp2=PCIN>>17  opr=+  inp1=P  carry=CIN  dbl_ovrd=off  block_type=constant
  Constant1 : xbsIndex_r4/Constant  const=0  gui_display_data_type=Fixed-point  arith_type=Unsigned  n_bits=1  bin_pt=0  preci_type=Single  exp_width=8  frac_width=24  explicit_period=off  period=1  equ=P=C  opselect=C  inp2=PCIN>>17  opr=+  inp1=P  carry=CIN  dbl_ovrd=off  block_type=constant
  Delay : xbsIndex_r4/Delay  rst=off  infoeditControl=Selection of Reset will increase slice count due to use of real FFs and instead of SRLs  en=off  latency=3  dbl_ovrd=off  reg_retiming=off  block_type=delay
  Down Sample1 : xbsIndex_r4/Down Sample  sample_ratio=n_ch/n_ovs  sample_phase="Last Value of Frame  (most efficient)"  en=off  latency=1  dbl_ovrd=off  block_type=dsamp
  Down Sample2 : xbsIndex_r4/Down Sample  sample_ratio=n_ch/n_ovs  sample_phase="Last Value of Frame  (most efficient)"  en=off  latency=1  dbl_ovrd=off  block_type=dsamp
  Register : xbsIndex_r4/Register  init=0  rst=off  en=on  dbl_ovrd=off  block_type=register
  Register1 : xbsIndex_r4/Register  init=0  rst=off  en=on  dbl_ovrd=off  block_type=register
  Relational : xbsIndex_r4/Relational  mode=a=b  en=off  latency=1  dbl_ovrd=off  block_type=relational
  Relational1 : xbsIndex_r4/Relational  mode=a=b  en=off  latency=1  dbl_ovrd=off  block_type=relational
  dout_ch0 : Outport
  dout_ch1 : Outport  Port=2
  ch_out : Outport  Port=3
  wires:
  Constant/1 -> Relational/2
  Constant1/1 -> Relational1/2
  Relational/1 -> Register/2
  Relational1/1 -> Register1/2
  din/1 -> Register/1, Register1/1
  Register/1 -> Down Sample2/1
  ch_in/1 -> Relational/1, Relational1/1, Delay/1
  Register1/1 -> Down Sample1/1
  Down Sample2/1 -> dout_ch0/1
  Delay/1 -> ch_out/1
  Down Sample1/1 -> dout_ch1/1

== system ddc_bpm_476_066/FOFB_amp/fofb_amp1/FOFB_amp/TDDM_fofb_cic1/TDDM_fofb_cic1_i ==
  din : Inport
  ch_in : Inport  Port=2
  Constant : xbsIndex_r4/Constant  const=1  gui_display_data_type=Fixed-point  arith_type=Unsigned  n_bits=1  bin_pt=0  preci_type=Single  exp_width=8  frac_width=24  explicit_period=off  period=1  equ=P=C  opselect=C  inp2=PCIN>>17  opr=+  inp1=P  carry=CIN  dbl_ovrd=off  block_type=constant
  Constant1 : xbsIndex_r4/Constant  const=0  gui_display_data_type=Fixed-point  arith_type=Unsigned  n_bits=1  bin_pt=0  preci_type=Single  exp_width=8  frac_width=24  explicit_period=off  period=1  equ=P=C  opselect=C  inp2=PCIN>>17  opr=+  inp1=P  carry=CIN  dbl_ovrd=off  block_type=constant
  Delay : xbsIndex_r4/Delay  rst=off  infoeditControl=Selection of Reset will increase slice count due to use of real FFs and instead of SRLs  en=off  latency=3  dbl_ovrd=off  reg_retiming=off  block_type=delay
  Down Sample1 : xbsIndex_r4/Down Sample  sample_ratio=n_ch/n_ovs  sample_phase="Last Value of Frame  (most efficient)"  en=off  latency=1  dbl_ovrd=off  block_type=dsamp
  Down Sample2 : xbsIndex_r4/Down Sample  sample_ratio=n_ch/n_ovs  sample_phase="Last Value of Frame  (most efficient)"  en=off  latency=1  dbl_ovrd=off  block_type=dsamp
  Register : xbsIndex_r4/Register  init=0  rst=off  en=on  dbl_ovrd=off  block_type=register
  Register1 : xbsIndex_r4/Register  init=0  rst=off  en=on  dbl_ovrd=off  block_type=register
  Relational : xbsIndex_r4/Relational  mode=a=b  en=off  latency=1  dbl_ovrd=off  block_type=relational
  Relational1 : xbsIndex_r4/Relational  mode=a=b  en=off  latency=1  dbl_ovrd=off  block_type=relational
  dout_ch0 : Outport
  dout_ch1 : Outport  Port=2
  ch_out : Outport  Port=3
  wires:
  Constant/1 -> Relational/2
  Constant1/1 -> Relational1/2
  Relational/1 -> Register/2
  Relational1/1 -> Register1/2
  din/1 -> Register/1, Register1/1
  Register/1 -> Down Sample2/1
  ch_in/1 -> Relational/1, Relational1/1, Delay/1
  Register1/1 -> Down Sample1/1
  Down Sample2/1 -> dout_ch0/1
  Delay/1 -> ch_out/1
  Down Sample1/1 -> dout_ch1/1

== system ddc_bpm_476_066/FOFB_amp/fofb_amp1/FOFB_amp/TDDM_fofb_cic1/TDDM_fofb_cic1_q ==
  din : Inport
  ch_in : Inport  Port=2
  Constant : xbsIndex_r4/Constant  const=1  gui_display_data_type=Fixed-point  arith_type=Unsigned  n_bits=1  bin_pt=0  preci_type=Single  exp_width=8  frac_width=24  explicit_period=off  period=1  equ=P=C  opselect=C  inp2=PCIN>>17  opr=+  inp1=P  carry=CIN  dbl_ovrd=off  block_type=constant
  Constant1 : xbsIndex_r4/Constant  const=0  gui_display_data_type=Fixed-point  arith_type=Unsigned  n_bits=1  bin_pt=0  preci_type=Single  exp_width=8  frac_width=24  explicit_period=off  period=1  equ=P=C  opselect=C  inp2=PCIN>>17  opr=+  inp1=P  carry=CIN  dbl_ovrd=off  block_type=constant
  Delay : xbsIndex_r4/Delay  rst=off  infoeditControl=Selection of Reset will increase slice count due to use of real FFs and instead of SRLs  en=off  latency=3  dbl_ovrd=off  reg_retiming=off  block_type=delay
  Down Sample1 : xbsIndex_r4/Down Sample  sample_ratio=n_ch/n_ovs  sample_phase="Last Value of Frame  (most efficient)"  en=off  latency=1  dbl_ovrd=off  block_type=dsamp
  Down Sample2 : xbsIndex_r4/Down Sample  sample_ratio=n_ch/n_ovs  sample_phase="Last Value of Frame  (most efficient)"  en=off  latency=1  dbl_ovrd=off  block_type=dsamp
  Register : xbsIndex_r4/Register  init=0  rst=off  en=on  dbl_ovrd=off  block_type=register
  Register1 : xbsIndex_r4/Register  init=0  rst=off  en=on  dbl_ovrd=off  block_type=register
  Relational : xbsIndex_r4/Relational  mode=a=b  en=off  latency=1  dbl_ovrd=off  block_type=relational
  Relational1 : xbsIndex_r4/Relational  mode=a=b  en=off  latency=1  dbl_ovrd=off  block_type=relational
  dout_ch0 : Outport
  dout_ch1 : Outport  Port=2
  ch_out : Outport  Port=3
  wires:
  Constant/1 -> Relational/2
  Constant1/1 -> Relational1/2
  Relational/1 -> Register/2
  Relational1/1 -> Register1/2
  din/1 -> Register/1, Register1/1
  Register/1 -> Down Sample2/1
  ch_in/1 -> Relational/1, Relational1/1, Delay/1
  Register1/1 -> Down Sample1/1
  Down Sample2/1 -> dout_ch0/1
  Delay/1 -> ch_out/1
  Down Sample1/1 -> dout_ch1/1

== system ddc_bpm_476_066/FOFB_amp/fofb_amp1/FOFB_amp/cic_fofb/Reg ==
  din : Inport
  en : Inport  Port=2
  Convert : xbsIndex_r4/Convert  gui_display_data_type=Fixed-point  arith_type="Signed  (2's comp)"  n_bits=25  bin_pt=23  float_type=Single  exp_bits=8  fraction_bits=24  quantization="Round  (unbiased: +/- Inf)"  overflow=Flag as error  en=off  latency=0  dbl_ovrd=off  pipeline=off  block_type=convert
  Register : xbsIndex_r4/Register  init=0  rst=off  en=on  dbl_ovrd=off  block_type=register
      settings: xl_area=[0, 0, 0, 0, 0, 0, 0]  block_version=VER_STRING_GOES_HERE
  Register1 : xbsIndex_r4/Register  init=0  rst=off  en=off  dbl_ovrd=off  block_type=register
      settings: xl_area=[0, 0, 0, 0, 0, 0, 0]  block_version=VER_STRING_GOES_HERE
  Reinterpret1 : xbsIndex_r4/Reinterpret  force_arith_type=on  arith_type="Signed  (2's comp)"  force_bin_pt=on  bin_pt=77  block_type=cast
      settings: block_version=VER_STRING_GOES_HERE
  dout : Outport
  valid_out : Outport  Port=2
  wires:
  Register/1 -> dout/1
  en/1 -> Register/2, Register1/1
  din/1 -> Reinterpret1/1
  Reinterpret1/1 -> Convert/1
  Register1/1 -> valid_out/1
  Convert/1 -> Register/1

== system ddc_bpm_476_066/FOFB_amp/fofb_amp1/FOFB_amp/cic_fofb/Reg1 ==
  din : Inport
  en : Inport  Port=2
  Convert : xbsIndex_r4/Convert  gui_display_data_type=Fixed-point  arith_type="Signed  (2's comp)"  n_bits=25  bin_pt=23  float_type=Single  exp_bits=8  fraction_bits=24  quantization="Round  (unbiased: +/- Inf)"  overflow=Flag as error  en=off  latency=0  dbl_ovrd=off  pipeline=off  block_type=convert
  Register : xbsIndex_r4/Register  init=0  rst=off  en=on  dbl_ovrd=off  block_type=register
      settings: xl_area=[0, 0, 0, 0, 0, 0, 0]  block_version=VER_STRING_GOES_HERE
  Register1 : xbsIndex_r4/Register  init=0  rst=off  en=off  dbl_ovrd=off  block_type=register
      settings: xl_area=[0, 0, 0, 0, 0, 0, 0]  block_version=VER_STRING_GOES_HERE
  Reinterpret2 : xbsIndex_r4/Reinterpret  force_arith_type=on  arith_type="Signed  (2's comp)"  force_bin_pt=on  bin_pt=77  block_type=cast
      settings: block_version=VER_STRING_GOES_HERE
  dout : Outport
  valid_out : Outport  Port=2
  wires:
  Register/1 -> dout/1
  en/1 -> Register/2, Register1/1
  din/1 -> Reinterpret2/1
  Reinterpret2/1 -> Convert/1
  Register1/1 -> valid_out/1
  Convert/1 -> Register/1

== system ddc_bpm_476_066/TBT_amp/TBT_amp0/TBT_CORDIC/TDDM_tbt_cordic/TDDM_tbt_cordic ==
  din : Inport
  ch_in : Inport  Port=2
  Constant : xbsIndex_r4/Constant  const=1  gui_display_data_type=Fixed-point  arith_type=Unsigned  n_bits=1  bin_pt=0  preci_type=Single  exp_width=8  frac_width=24  explicit_period=off  period=1  equ=P=C  opselect=C  inp2=PCIN>>17  opr=+  inp1=P  carry=CIN  dbl_ovrd=off  block_type=constant
  Constant1 : xbsIndex_r4/Constant  const=0  gui_display_data_type=Fixed-point  arith_type=Unsigned  n_bits=1  bin_pt=0  preci_type=Single  exp_width=8  frac_width=24  explicit_period=off  period=1  equ=P=C  opselect=C  inp2=PCIN>>17  opr=+  inp1=P  carry=CIN  dbl_ovrd=off  block_type=constant
  Delay : xbsIndex_r4/Delay  rst=off  infoeditControl=Selection of Reset will increase slice count due to use of real FFs and instead of SRLs  en=off  latency=3  dbl_ovrd=off  reg_retiming=off  block_type=delay
  Down Sample1 : xbsIndex_r4/Down Sample  sample_ratio=n_ch/n_ovs  sample_phase="Last Value of Frame  (most efficient)"  en=off  latency=1  dbl_ovrd=off  block_type=dsamp
  Down Sample2 : xbsIndex_r4/Down Sample  sample_ratio=n_ch/n_ovs  sample_phase="Last Value of Frame  (most efficient)"  en=off  latency=1  dbl_ovrd=off  block_type=dsamp
  Register : xbsIndex_r4/Register  init=0  rst=off  en=on  dbl_ovrd=off  block_type=register
  Register1 : xbsIndex_r4/Register  init=0  rst=off  en=on  dbl_ovrd=off  block_type=register
  Relational : xbsIndex_r4/Relational  mode=a=b  en=off  latency=1  dbl_ovrd=off  block_type=relational
  Relational1 : xbsIndex_r4/Relational  mode=a=b  en=off  latency=1  dbl_ovrd=off  block_type=relational
  dout_ch0 : Outport
  dout_ch1 : Outport  Port=2
  ch_out : Outport  Port=3
  wires:
  Constant/1 -> Relational/2
  Constant1/1 -> Relational1/2
  Relational/1 -> Register/2
  Relational1/1 -> Register1/2
  din/1 -> Register/1, Register1/1
  Register/1 -> Down Sample2/1
  ch_in/1 -> Relational/1, Relational1/1, Delay/1
  Register1/1 -> Down Sample1/1
  Down Sample2/1 -> dout_ch0/1
  Delay/1 -> ch_out/1
  Down Sample1/1 -> dout_ch1/1

== system ddc_bpm_476_066/TBT_amp/TBT_amp0/TBT_CORDIC/TDDM_tbt_cordic/TDDM_tbt_cordic1 ==
  din : Inport
  ch_in : Inport  Port=2
  Constant : xbsIndex_r4/Constant  const=1  gui_display_data_type=Fixed-point  arith_type=Unsigned  n_bits=1  bin_pt=0  preci_type=Single  exp_width=8  frac_width=24  explicit_period=off  period=1  equ=P=C  opselect=C  inp2=PCIN>>17  opr=+  inp1=P  carry=CIN  dbl_ovrd=off  block_type=constant
  Constant1 : xbsIndex_r4/Constant  const=0  gui_display_data_type=Fixed-point  arith_type=Unsigned  n_bits=1  bin_pt=0  preci_type=Single  exp_width=8  frac_width=24  explicit_period=off  period=1  equ=P=C  opselect=C  inp2=PCIN>>17  opr=+  inp1=P  carry=CIN  dbl_ovrd=off  block_type=constant
  Delay : xbsIndex_r4/Delay  rst=off  infoeditControl=Selection of Reset will increase slice count due to use of real FFs and instead of SRLs  en=off  latency=3  dbl_ovrd=off  reg_retiming=off  block_type=delay
  Down Sample1 : xbsIndex_r4/Down Sample  sample_ratio=n_ch/n_ovs  sample_phase="Last Value of Frame  (most efficient)"  en=off  latency=1  dbl_ovrd=off  block_type=dsamp
  Down Sample2 : xbsIndex_r4/Down Sample  sample_ratio=n_ch/n_ovs  sample_phase="Last Value of Frame  (most efficient)"  en=off  latency=1  dbl_ovrd=off  block_type=dsamp
  Register : xbsIndex_r4/Register  init=0  rst=off  en=on  dbl_ovrd=off  block_type=register
  Register1 : xbsIndex_r4/Register  init=0  rst=off  en=on  dbl_ovrd=off  block_type=register
  Relational : xbsIndex_r4/Relational  mode=a=b  en=off  latency=1  dbl_ovrd=off  block_type=relational
  Relational1 : xbsIndex_r4/Relational  mode=a=b  en=off  latency=1  dbl_ovrd=off  block_type=relational
  dout_ch0 : Outport
  dout_ch1 : Outport  Port=2
  ch_out : Outport  Port=3
  wires:
  Constant/1 -> Relational/2
  Constant1/1 -> Relational1/2
  Relational/1 -> Register/2
  Relational1/1 -> Register1/2
  din/1 -> Register/1, Register1/1
  Register/1 -> Down Sample2/1
  ch_in/1 -> Relational/1, Relational1/1, Delay/1
  Register1/1 -> Down Sample1/1
  Down Sample2/1 -> dout_ch0/1
  Delay/1 -> ch_out/1
  Down Sample1/1 -> dout_ch1/1
